simulink subsystem "MotorsG31"  (R2022b)
settings: Solver=VariableStepAuto  StartTime=0.0  StopTime=10.0  RelTol=1e-3
libraries: arduinolib x6, simulink x2
settings Model: Creator=dar.io  LastModifiedBy=dar.io

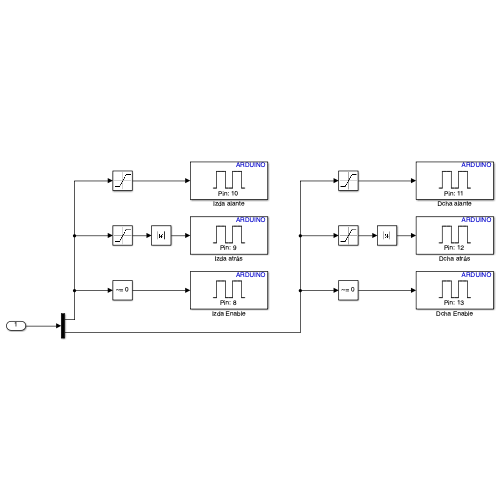
[thumbnail: Simulink's stored preview of the top-level diagram]
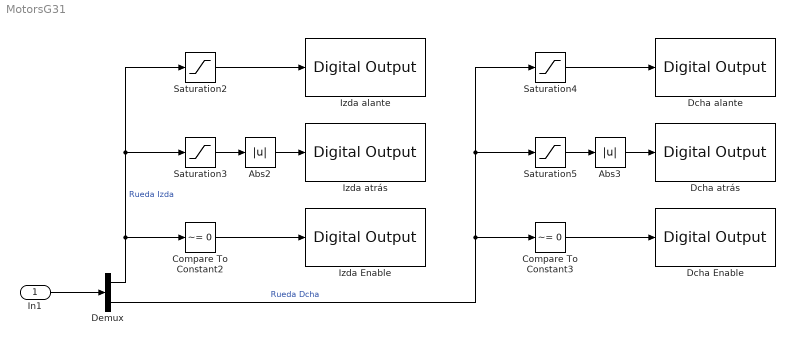
== system MotorsG31 ==
  In1 : Inport  OutDataTypeStr=int16
  Abs2 : Abs  SaturateOnIntegerOverflow=off
  Abs3 : Abs  SaturateOnIntegerOverflow=off
  Compare To Constant2 : simulink/Logic and Bit Operations/Compare To Constant  relop=~=  const=0  OutDataTypeStr=boolean
  Compare To Constant3 : simulink/Logic and Bit Operations/Compare To Constant  relop=~=  const=0  OutDataTypeStr=boolean
  Dcha Enable : arduinolib/Digital Output  pinNumber=13  Direction=output  blockPlatform=arduino
  Dcha alante : arduinolib/Digital Output  pinNumber=11  Direction=output  blockPlatform=arduino
  Dcha atrás : arduinolib/Digital Output  pinNumber=12  Direction=output  blockPlatform=arduino
  Demux : Demux  Outputs=2
  Izda Enable : arduinolib/Digital Output  pinNumber=8  Direction=output  blockPlatform=arduino
  Izda alante : arduinolib/Digital Output  pinNumber=10  Direction=output  blockPlatform=arduino
  Izda atrás : arduinolib/Digital Output  pinNumber=9  Direction=output  blockPlatform=arduino
  Saturation2 : Saturate  UpperLimit=255  LowerLimit=0
  Saturation3 : Saturate  UpperLimit=0  LowerLimit=-255
  Saturation4 : Saturate  UpperLimit=255  LowerLimit=0
  Saturation5 : Saturate  UpperLimit=0  LowerLimit=-255
  wires:
  Saturation2/1 -> Izda alante/1
  Abs2/1 -> Izda atrás/1
  Saturation3/1 -> Abs2/1
  Compare To Constant2/1 -> Izda Enable/1
  Demux/2 -> Compare To Constant3/1, Saturation5/1, Saturation4/1  "Rueda Dcha"
  Abs3/1 -> Dcha atrás/1
  Demux/1 -> Compare To Constant2/1, Saturation3/1, Saturation2/1  "Rueda Izda"
  Saturation4/1 -> Dcha alante/1
  Compare To Constant3/1 -> Dcha Enable/1
  Saturation5/1 -> Abs3/1
  In1/1 -> Demux/1
